simulink model "ThdRwRtStFwdBkwdTrgtPosSelc"  (R2018b)
settings: Solver=FixedStepDiscrete  StartTime=0.0  StopTime=10.0  FixedStep=0.01  RelTol=1e-3
undefined symbols (not defined in the file or in its folder): KeSMSw6sAcsEntryThdRwRtStFrwdBkwdPos_Val, KeSMSw6sAcsEntryThdRwRtStFrwdBkwdPosMax_Val, KeSMSw6sAcsEntryThdRwRtStFrwdBkwdPosMin_Val, KeSMSw6sFamilyMdThdRwRtStFrwdBkwdPos_Val, KeSMSw6sFamilyMdThdRwRtStFrwdBkwdPosMax_Val, KeSMSw6sFamilyMdThdRwRtStFrwdBkwdPosMin_Val, KeSMSw6sFamilyRMdThdRwRtStFrwdBkwdPos_Val, KeSMSw6sFamilyRMdThdRwRtStFrwdBkwdPosMax_Val, KeSMSw6sFamilyRMdThdRwRtStFrwdBkwdPosMin_Val, KeSMSw6sLugThdRwRtStFrwdBkwdPos_Val, KeSMSw6sLugThdRwRtStFrwdBkwdPosMax_Val, KeSMSw6sLugThdRwRtStFrwdBkwdPosMin_Val, KeSMSw6sVIPThdRwRtStFrwdBkwdPos_Val, KeSMSw6sVIPThdRwRtStFrwdBkwdPosMax_Val, KeSMSw6sVIPThdRwRtStFrwdBkwdPosMin_Val, KeSMSwAcsEntryThdRwRtStFrwdBkwdPos_Val, KeSMSwAcsEntryThdRwRtStFrwdBkwdPosMax_Val, KeSMSwAcsEntryThdRwRtStFrwdBkwdPosMin_Val, KeSMSwFamilyMdThdRwRtStFrwdBkwdPos_Val, KeSMSwFamilyMdThdRwRtStFrwdBkwdPosMax_Val, KeSMSwFamilyMdThdRwRtStFrwdBkwdPosMin_Val, KeSMSwFamilyRMdThdRwRtStFrwdBkwdPos_Val, KeSMSwFamilyRMdThdRwRtStFrwdBkwdPosMax_Val, KeSMSwFamilyRMdThdRwRtStFrwdBkwdPosMin_Val, KeSMSwLugThdRwRtStFrwdBkwdPos_Val, KeSMSwLugThdRwRtStFrwdBkwdPosMax_Val, KeSMSwLugThdRwRtStFrwdBkwdPosMin_Val, KeSMSwVIPThdRwRtStFrwdBkwdPos_Val, KeSMSwVIPThdRwRtStFrwdBkwdPosMax_Val, KeSMSwVIPThdRwRtStFrwdBkwdPosMin_Val
libraries: TrgtPosSelcLib x6
settings Model: Creator=sn2xws  LastModifiedBy=sn2xws
settings Model: ModifiedHistory=|
  | V2.1.0 Bug 540874 将外部标定改为固定值0
  | 2024.7.8 V3.0.0 557模式流程V1.9
settings DataIOCC: SaveFormat=StructureWithTime
settings OptimizationCC: DefaultParameterBehavior=Inlined  EnhancedBackFolding=on  PassReuseOutputArgsAs=Individual arguments  ZeroExternalMemoryAtStartup=off  ZeroInternalMemoryAtStartup=off  OptimizeBlockOrder=speed  DifferentSizesBufferReuse=on  OptimizationCustomize=off
settings DebuggingCC: ParameterTunabilityLossMsg=error
settings SFSimCC: MATLABDynamicMemAlloc=off
settings RTWCC: SystemTargetFile=autosar.tlc  GenCodeOnly=on  TemplateMakefile=ert_default_tmf  Description=AUTOSAR  GenerateReport=on  IncludeHyperlinkInReport=on  LaunchReport=on  GenerateTraceInfo=on  GenerateTraceReport=on  GenerateTraceReportSl=on  GenerateTraceReportSf=on  GenerateTraceReportEml=on  GenerateCodeMetricsReport=on
settings CodeAppCC: ForceParamTrailComments=on  IgnoreCustomStorageClasses=off  OperatorAnnotations=on  SimulinkDataObjDesc=on  SFDataObjDesc=on  InsertBlockDesc=on
settings STFCustomTargetCC: TargetLangStandard=C99 (ISO)  MultiwordLength=256  ParMdlRefBuildCompliant=on  CompOptLevelCompliant=on  IncludeMdlTerminateFcn=off  CombineOutputUpdateFcns=on  SuppressErrorStatus=on  ERTCustomFileBanners=on  SupportNonFinite=off  SupportComplex=off  SupportContinuousTime=off  SupportNonInlinedSFcns=off  RemoveResetFunc=on  MATLABClassNameForMDSCustomization=Simulink.SoftwareTarget.ERTCustomization  AutosarCompliant=on  UseToolchainInfoCompliant=on  LookupTableObjectStructAxisOrder=2,1,3,4,...  LUTObjectStructOrderEvenSpacing=Size,Table,Breakpoints  SystemTargetFile=autosar.tlc
settings ERTTargetCC: TargetLangStandard=C99 (ISO)  ConcurrentExecutionCompliant=off  IncludeMdlTerminateFcn=off  SuppressErrorStatus=on  SupportNonFinite=off  SupportComplex=off  ModelStepFunctionPrototypeControlCompliant=off  CPPClassGenCompliant=off  AutosarCompliant=on  LookupTableObjectStructAxisOrder=2,1,3,4,...  LUTObjectStructOrderEvenSpacing=Size,Table,Breakpoints  InlinedParameterPlacement=NonHierarchical  ERTCustomFileTemplate=example_file_process.tlc  ERTFilePackagingFormat=Compact

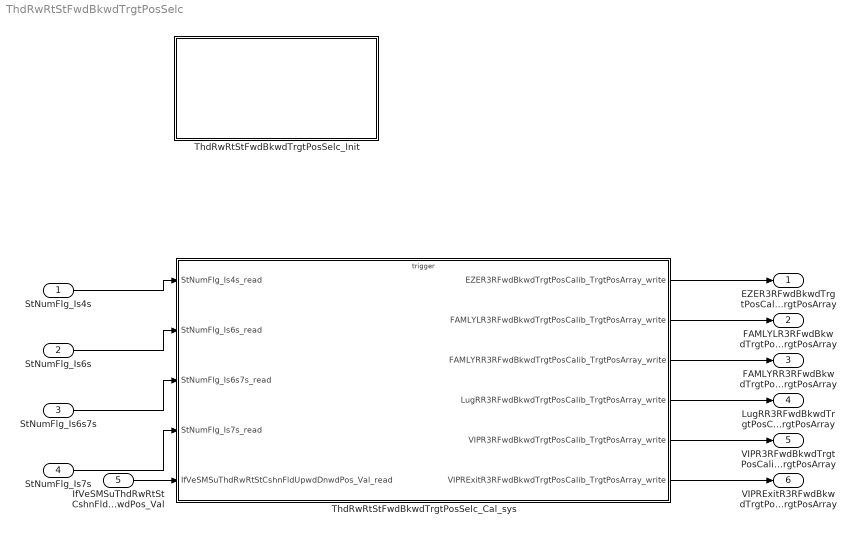
== system ThdRwRtStFwdBkwdTrgtPosSelc ==
  StNumFlg_Is4s : Inport  OutDataTypeStr=boolean  PortDimensions=1
  StNumFlg_Is6s : Inport  Port=2  OutDataTypeStr=boolean  PortDimensions=1
  StNumFlg_Is6s7s : Inport  Port=3  OutDataTypeStr=boolean  PortDimensions=1
  StNumFlg_Is7s : Inport  Port=4  OutDataTypeStr=boolean  PortDimensions=1
  IfVeSMSuThdRwRtStCshnFldUpwdDnwdPos_Val : Inport  Port=5  OutDataTypeStr=uint16  PortDimensions=1
  ThdRwRtStFwdBkwdTrgtPosSelc_Cal_sys : Subsystem
  ThdRwRtStFwdBkwdTrgtPosSelc_Init : Subsystem
  EZER3RFwdBkwdTrgtPosCalib_TrgtPosArray : Outport  Description=|  OutDataTypeStr=uint16  PortDimensions=3
      | 0:Pos
      | 1:Max
      | 2:Min
  FAMLYLR3RFwdBkwdTrgtPosCalib_TrgtPosArray : Outport  Description=|  Port=2  OutDataTypeStr=uint16  PortDimensions=3
      | 0:Pos
      | 1:Max
      | 2:Min
  FAMLYRR3RFwdBkwdTrgtPosCalib_TrgtPosArray : Outport  Description=|  Port=3  OutDataTypeStr=uint16  PortDimensions=3
      | 0:Pos
      | 1:Max
      | 2:Min
  LugRR3RFwdBkwdTrgtPosCalib_TrgtPosArray : Outport  Description=|  Port=4  OutDataTypeStr=uint16  PortDimensions=3
      | 0:Pos
      | 1:Max
      | 2:Min
  VIPR3RFwdBkwdTrgtPosCalib_TrgtPosArray : Outport  Description=|  Port=5  OutDataTypeStr=uint16  PortDimensions=3
      | 0:Pos
      | 1:Max
      | 2:Min
  VIPRExitR3RFwdBkwdTrgtPosCalib_TrgtPosArray : Outport  Description=|  Port=6  OutDataTypeStr=uint16  PortDimensions=3
      | 0:Pos
      | 1:Max
      | 2:Min
  wires:
  StNumFlg_Is4s/1 -> ThdRwRtStFwdBkwdTrgtPosSelc_Cal_sys/1(StNumFlg_Is4s_read)
  StNumFlg_Is6s/1 -> ThdRwRtStFwdBkwdTrgtPosSelc_Cal_sys/2(StNumFlg_Is6s_read)
  StNumFlg_Is6s7s/1 -> ThdRwRtStFwdBkwdTrgtPosSelc_Cal_sys/3(StNumFlg_Is6s7s_read)
  StNumFlg_Is7s/1 -> ThdRwRtStFwdBkwdTrgtPosSelc_Cal_sys/4(StNumFlg_Is7s_read)
  ThdRwRtStFwdBkwdTrgtPosSelc_Cal_sys/1(EZER3RFwdBkwdTrgtPosCalib_TrgtPosArray_write) -> EZER3RFwdBkwdTrgtPosCalib_TrgtPosArray/1
  ThdRwRtStFwdBkwdTrgtPosSelc_Cal_sys/2(FAMLYLR3RFwdBkwdTrgtPosCalib_TrgtPosArray_write) -> FAMLYLR3RFwdBkwdTrgtPosCalib_TrgtPosArray/1
  ThdRwRtStFwdBkwdTrgtPosSelc_Cal_sys/3(FAMLYRR3RFwdBkwdTrgtPosCalib_TrgtPosArray_write) -> FAMLYRR3RFwdBkwdTrgtPosCalib_TrgtPosArray/1
  ThdRwRtStFwdBkwdTrgtPosSelc_Cal_sys/4(LugRR3RFwdBkwdTrgtPosCalib_TrgtPosArray_write) -> LugRR3RFwdBkwdTrgtPosCalib_TrgtPosArray/1
  ThdRwRtStFwdBkwdTrgtPosSelc_Cal_sys/5(VIPR3RFwdBkwdTrgtPosCalib_TrgtPosArray_write) -> VIPR3RFwdBkwdTrgtPosCalib_TrgtPosArray/1
  ThdRwRtStFwdBkwdTrgtPosSelc_Cal_sys/6(VIPRExitR3RFwdBkwdTrgtPosCalib_TrgtPosArray_write) -> VIPRExitR3RFwdBkwdTrgtPosCalib_TrgtPosArray/1
  IfVeSMSuThdRwRtStCshnFldUpwdDnwdPos_Val/1 -> ThdRwRtStFwdBkwdTrgtPosSelc_Cal_sys/5(IfVeSMSuThdRwRtStCshnFldUpwdDnwdPos_Val_read)

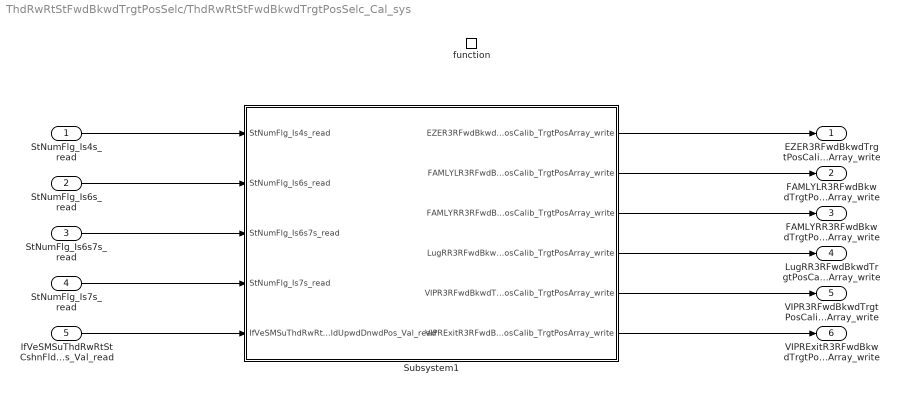
== system ThdRwRtStFwdBkwdTrgtPosSelc/ThdRwRtStFwdBkwdTrgtPosSelc_Cal_sys ==
  StNumFlg_Is4s_read : Inport
  StNumFlg_Is6s_read : Inport  Port=2
  StNumFlg_Is6s7s_read : Inport  Port=3
  StNumFlg_Is7s_read : Inport  Port=4
  IfVeSMSuThdRwRtStCshnFldUpwdDnwdPos_Val_read : Inport  Port=5
  function : TriggerPort  TriggerType=function-call  IsSimulinkFunction=on  FunctionName=ThdRwRtStFwdBkwdTrgtPosSelc_Cal  VariantControl=(inherit)
  Subsystem1 : Subsystem
  EZER3RFwdBkwdTrgtPosCalib_TrgtPosArray_write : Outport
      settings: EnsureOutportIsVirtual=on
  FAMLYLR3RFwdBkwdTrgtPosCalib_TrgtPosArray_write : Outport  Port=2
      settings: EnsureOutportIsVirtual=on
  FAMLYRR3RFwdBkwdTrgtPosCalib_TrgtPosArray_write : Outport  Port=3
      settings: EnsureOutportIsVirtual=on
  LugRR3RFwdBkwdTrgtPosCalib_TrgtPosArray_write : Outport  Port=4
      settings: EnsureOutportIsVirtual=on
  VIPR3RFwdBkwdTrgtPosCalib_TrgtPosArray_write : Outport  Port=5
      settings: EnsureOutportIsVirtual=on
  VIPRExitR3RFwdBkwdTrgtPosCalib_TrgtPosArray_write : Outport  Port=6
      settings: EnsureOutportIsVirtual=on
  wires:
  Subsystem1/2(FAMLYLR3RFwdBkwdTrgtPosCalib_TrgtPosArray_write) -> FAMLYLR3RFwdBkwdTrgtPosCalib_TrgtPosArray_write/1
  Subsystem1/1(EZER3RFwdBkwdTrgtPosCalib_TrgtPosArray_write) -> EZER3RFwdBkwdTrgtPosCalib_TrgtPosArray_write/1
  Subsystem1/3(FAMLYRR3RFwdBkwdTrgtPosCalib_TrgtPosArray_write) -> FAMLYRR3RFwdBkwdTrgtPosCalib_TrgtPosArray_write/1
  Subsystem1/4(LugRR3RFwdBkwdTrgtPosCalib_TrgtPosArray_write) -> LugRR3RFwdBkwdTrgtPosCalib_TrgtPosArray_write/1
  Subsystem1/5(VIPR3RFwdBkwdTrgtPosCalib_TrgtPosArray_write) -> VIPR3RFwdBkwdTrgtPosCalib_TrgtPosArray_write/1
  StNumFlg_Is4s_read/1 -> Subsystem1/1(StNumFlg_Is4s_read)
  StNumFlg_Is6s_read/1 -> Subsystem1/2(StNumFlg_Is6s_read)
  StNumFlg_Is6s7s_read/1 -> Subsystem1/3(StNumFlg_Is6s7s_read)
  StNumFlg_Is7s_read/1 -> Subsystem1/4(StNumFlg_Is7s_read)
  Subsystem1/6(VIPRExitR3RFwdBkwdTrgtPosCalib_TrgtPosArray_write) -> VIPRExitR3RFwdBkwdTrgtPosCalib_TrgtPosArray_write/1
  IfVeSMSuThdRwRtStCshnFldUpwdDnwdPos_Val_read/1 -> Subsystem1/5(IfVeSMSuThdRwRtStCshnFldUpwdDnwdPos_Val_read)

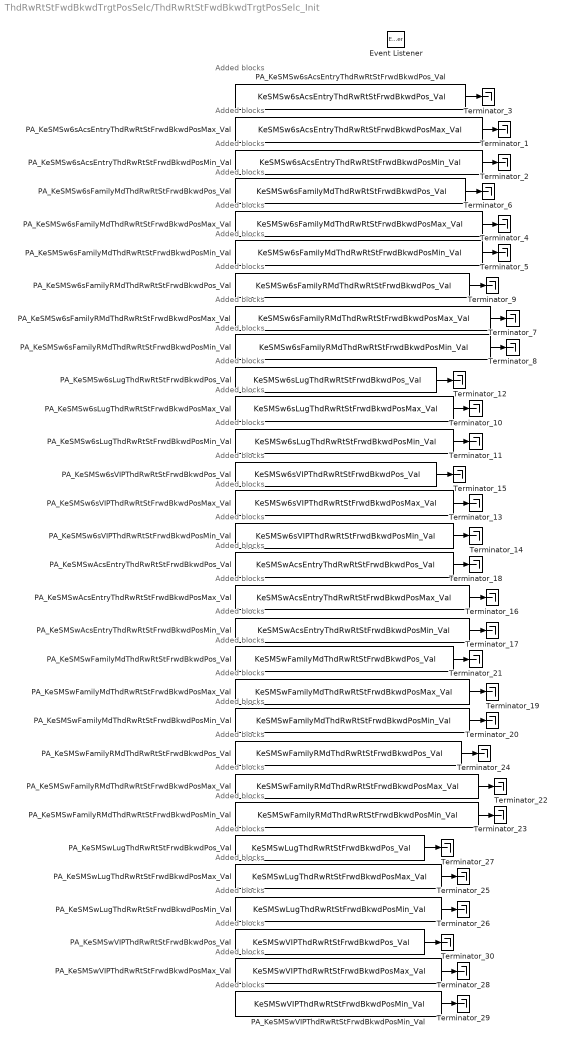
== system ThdRwRtStFwdBkwdTrgtPosSelc/ThdRwRtStFwdBkwdTrgtPosSelc_Init ==
  note: Added blocks
  note: Added blocks
  note: Added blocks
  note: Added blocks
  note: Added blocks
  note: Added blocks
  note: Added blocks
  note: Added blocks
  note: Added blocks
  note: Added blocks
  note: Added blocks
  note: Added blocks
  note: Added blocks
  note: Added blocks
  note: Added blocks
  note: Added blocks
  note: Added blocks
  note: Added blocks
  note: Added blocks
  note: Added blocks
  note: Added blocks
  note: Added blocks
  note: Added blocks
  note: Added blocks
  note: Added blocks
  note: Added blocks
  note: Added blocks
  note: Added blocks
  note: Added blocks
  note: Added blocks
  Event Listener : EventListener  EventName=reset
  PA_KeSMSw6sAcsEntryThdRwRtStFrwdBkwdPosMax_Val : Constant  Value=KeSMSw6sAcsEntryThdRwRtStFrwdBkwdPosMax_Val
  PA_KeSMSw6sAcsEntryThdRwRtStFrwdBkwdPosMin_Val : Constant  Value=KeSMSw6sAcsEntryThdRwRtStFrwdBkwdPosMin_Val
  PA_KeSMSw6sAcsEntryThdRwRtStFrwdBkwdPos_Val : Constant  Value=KeSMSw6sAcsEntryThdRwRtStFrwdBkwdPos_Val
  PA_KeSMSw6sFamilyMdThdRwRtStFrwdBkwdPosMax_Val : Constant  Value=KeSMSw6sFamilyMdThdRwRtStFrwdBkwdPosMax_Val
  PA_KeSMSw6sFamilyMdThdRwRtStFrwdBkwdPosMin_Val : Constant  Value=KeSMSw6sFamilyMdThdRwRtStFrwdBkwdPosMin_Val
  PA_KeSMSw6sFamilyMdThdRwRtStFrwdBkwdPos_Val : Constant  Value=KeSMSw6sFamilyMdThdRwRtStFrwdBkwdPos_Val
  PA_KeSMSw6sFamilyRMdThdRwRtStFrwdBkwdPosMax_Val : Constant  Value=KeSMSw6sFamilyRMdThdRwRtStFrwdBkwdPosMax_Val
  PA_KeSMSw6sFamilyRMdThdRwRtStFrwdBkwdPosMin_Val : Constant  Value=KeSMSw6sFamilyRMdThdRwRtStFrwdBkwdPosMin_Val
  PA_KeSMSw6sFamilyRMdThdRwRtStFrwdBkwdPos_Val : Constant  Value=KeSMSw6sFamilyRMdThdRwRtStFrwdBkwdPos_Val
  PA_KeSMSw6sLugThdRwRtStFrwdBkwdPosMax_Val : Constant  Value=KeSMSw6sLugThdRwRtStFrwdBkwdPosMax_Val
  PA_KeSMSw6sLugThdRwRtStFrwdBkwdPosMin_Val : Constant  Value=KeSMSw6sLugThdRwRtStFrwdBkwdPosMin_Val
  PA_KeSMSw6sLugThdRwRtStFrwdBkwdPos_Val : Constant  Value=KeSMSw6sLugThdRwRtStFrwdBkwdPos_Val
  PA_KeSMSw6sVIPThdRwRtStFrwdBkwdPosMax_Val : Constant  Value=KeSMSw6sVIPThdRwRtStFrwdBkwdPosMax_Val
  PA_KeSMSw6sVIPThdRwRtStFrwdBkwdPosMin_Val : Constant  Value=KeSMSw6sVIPThdRwRtStFrwdBkwdPosMin_Val
  PA_KeSMSw6sVIPThdRwRtStFrwdBkwdPos_Val : Constant  Value=KeSMSw6sVIPThdRwRtStFrwdBkwdPos_Val
  PA_KeSMSwAcsEntryThdRwRtStFrwdBkwdPosMax_Val : Constant  Value=KeSMSwAcsEntryThdRwRtStFrwdBkwdPosMax_Val
  PA_KeSMSwAcsEntryThdRwRtStFrwdBkwdPosMin_Val : Constant  Value=KeSMSwAcsEntryThdRwRtStFrwdBkwdPosMin_Val
  PA_KeSMSwAcsEntryThdRwRtStFrwdBkwdPos_Val : Constant  Value=KeSMSwAcsEntryThdRwRtStFrwdBkwdPos_Val
  PA_KeSMSwFamilyMdThdRwRtStFrwdBkwdPosMax_Val : Constant  Value=KeSMSwFamilyMdThdRwRtStFrwdBkwdPosMax_Val
  PA_KeSMSwFamilyMdThdRwRtStFrwdBkwdPosMin_Val : Constant  Value=KeSMSwFamilyMdThdRwRtStFrwdBkwdPosMin_Val
  PA_KeSMSwFamilyMdThdRwRtStFrwdBkwdPos_Val : Constant  Value=KeSMSwFamilyMdThdRwRtStFrwdBkwdPos_Val
  PA_KeSMSwFamilyRMdThdRwRtStFrwdBkwdPosMax_Val : Constant  Value=KeSMSwFamilyRMdThdRwRtStFrwdBkwdPosMax_Val
  PA_KeSMSwFamilyRMdThdRwRtStFrwdBkwdPosMin_Val : Constant  Value=KeSMSwFamilyRMdThdRwRtStFrwdBkwdPosMin_Val
  PA_KeSMSwFamilyRMdThdRwRtStFrwdBkwdPos_Val : Constant  Value=KeSMSwFamilyRMdThdRwRtStFrwdBkwdPos_Val
  PA_KeSMSwLugThdRwRtStFrwdBkwdPosMax_Val : Constant  Value=KeSMSwLugThdRwRtStFrwdBkwdPosMax_Val
  PA_KeSMSwLugThdRwRtStFrwdBkwdPosMin_Val : Constant  Value=KeSMSwLugThdRwRtStFrwdBkwdPosMin_Val
  PA_KeSMSwLugThdRwRtStFrwdBkwdPos_Val : Constant  Value=KeSMSwLugThdRwRtStFrwdBkwdPos_Val
  PA_KeSMSwVIPThdRwRtStFrwdBkwdPosMax_Val : Constant  Value=KeSMSwVIPThdRwRtStFrwdBkwdPosMax_Val
  PA_KeSMSwVIPThdRwRtStFrwdBkwdPosMin_Val : Constant  Value=KeSMSwVIPThdRwRtStFrwdBkwdPosMin_Val
  PA_KeSMSwVIPThdRwRtStFrwdBkwdPos_Val : Constant  Value=KeSMSwVIPThdRwRtStFrwdBkwdPos_Val
  Terminator_{1..30} (30 alike) : Terminator
  wires:
  PA_KeSMSw6sAcsEntryThdRwRtStFrwdBkwdPosMax_Val/1 -> Terminator_1/1
  PA_KeSMSw6sAcsEntryThdRwRtStFrwdBkwdPosMin_Val/1 -> Terminator_2/1
  PA_KeSMSw6sAcsEntryThdRwRtStFrwdBkwdPos_Val/1 -> Terminator_3/1
  PA_KeSMSw6sFamilyMdThdRwRtStFrwdBkwdPosMax_Val/1 -> Terminator_4/1
  PA_KeSMSw6sFamilyMdThdRwRtStFrwdBkwdPosMin_Val/1 -> Terminator_5/1
  PA_KeSMSw6sFamilyMdThdRwRtStFrwdBkwdPos_Val/1 -> Terminator_6/1
  PA_KeSMSw6sFamilyRMdThdRwRtStFrwdBkwdPosMax_Val/1 -> Terminator_7/1
  PA_KeSMSw6sFamilyRMdThdRwRtStFrwdBkwdPosMin_Val/1 -> Terminator_8/1
  PA_KeSMSw6sFamilyRMdThdRwRtStFrwdBkwdPos_Val/1 -> Terminator_9/1
  PA_KeSMSw6sLugThdRwRtStFrwdBkwdPosMax_Val/1 -> Terminator_10/1
  PA_KeSMSw6sLugThdRwRtStFrwdBkwdPosMin_Val/1 -> Terminator_11/1
  PA_KeSMSw6sLugThdRwRtStFrwdBkwdPos_Val/1 -> Terminator_12/1
  PA_KeSMSw6sVIPThdRwRtStFrwdBkwdPosMax_Val/1 -> Terminator_13/1
  PA_KeSMSw6sVIPThdRwRtStFrwdBkwdPosMin_Val/1 -> Terminator_14/1
  PA_KeSMSw6sVIPThdRwRtStFrwdBkwdPos_Val/1 -> Terminator_15/1
  PA_KeSMSwAcsEntryThdRwRtStFrwdBkwdPosMax_Val/1 -> Terminator_16/1
  PA_KeSMSwAcsEntryThdRwRtStFrwdBkwdPosMin_Val/1 -> Terminator_17/1
  PA_KeSMSwAcsEntryThdRwRtStFrwdBkwdPos_Val/1 -> Terminator_18/1
  PA_KeSMSwFamilyMdThdRwRtStFrwdBkwdPosMax_Val/1 -> Terminator_19/1
  PA_KeSMSwFamilyMdThdRwRtStFrwdBkwdPosMin_Val/1 -> Terminator_20/1
  PA_KeSMSwFamilyMdThdRwRtStFrwdBkwdPos_Val/1 -> Terminator_21/1
  PA_KeSMSwFamilyRMdThdRwRtStFrwdBkwdPosMax_Val/1 -> Terminator_22/1
  PA_KeSMSwFamilyRMdThdRwRtStFrwdBkwdPosMin_Val/1 -> Terminator_23/1
  PA_KeSMSwFamilyRMdThdRwRtStFrwdBkwdPos_Val/1 -> Terminator_24/1
  PA_KeSMSwLugThdRwRtStFrwdBkwdPosMax_Val/1 -> Terminator_25/1
  PA_KeSMSwLugThdRwRtStFrwdBkwdPosMin_Val/1 -> Terminator_26/1
  PA_KeSMSwLugThdRwRtStFrwdBkwdPos_Val/1 -> Terminator_27/1
  PA_KeSMSwVIPThdRwRtStFrwdBkwdPosMax_Val/1 -> Terminator_28/1
  PA_KeSMSwVIPThdRwRtStFrwdBkwdPosMin_Val/1 -> Terminator_29/1
  PA_KeSMSwVIPThdRwRtStFrwdBkwdPos_Val/1 -> Terminator_30/1

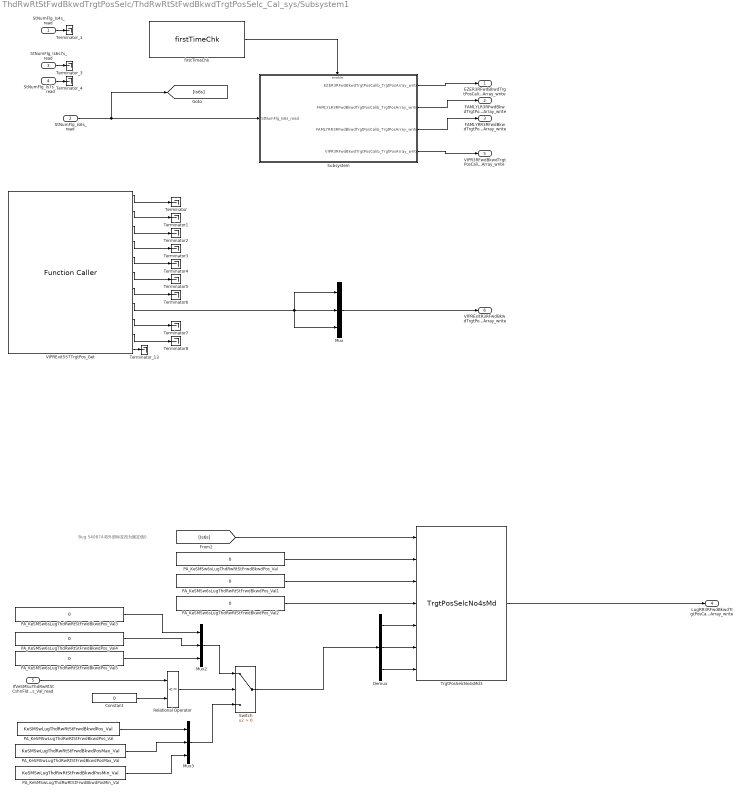
== system ThdRwRtStFwdBkwdTrgtPosSelc/ThdRwRtStFwdBkwdTrgtPosSelc_Cal_sys/Subsystem1 ==
  note: Bug 540874 将外部标定改为固定值0
  StNumFlg_Is4s_read : Inport
  StNumFlg_Is6s_read : Inport  Port=2
  StNumFlg_Is6s7s_read : Inport  Port=3
  StNumFlg_Is7s_read : Inport  Port=4
  IfVeSMSuThdRwRtStCshnFldUpwdDnwdPos_Val_read : Inport  Port=5
  Constant : Constant  Value=0  OutDataTypeStr=uint16
  Demux : Demux  Outputs=3
  Mux : Mux  Inputs=3
  Mux2 : Mux  Inputs=3
  Mux3 : Mux  Inputs=3
  PA_KeSMSw6sLugThdRwRtStFrwdBkwdPos_Val{,1..5} (6 alike) : Constant  Value=0  OutDataTypeStr=uint16
  PA_KeSMSwLugThdRwRtStFrwdBkwdPosMax_Val : Constant  Value=KeSMSwLugThdRwRtStFrwdBkwdPosMax_Val
  PA_KeSMSwLugThdRwRtStFrwdBkwdPosMin_Val : Constant  Value=KeSMSwLugThdRwRtStFrwdBkwdPosMin_Val
  PA_KeSMSwLugThdRwRtStFrwdBkwdPos_Val : Constant  Value=KeSMSwLugThdRwRtStFrwdBkwdPos_Val
  Relational Operator : RelationalOperator  Operator=<=  OutDataTypeStr=boolean  RndMeth=Simplest
  Subsystem : Subsystem
  Switch : Switch  Criteria=u2 > Threshold
  Terminator{,1..8} (9 alike) : Terminator
  Terminator_{1,3..4,13} (4 alike) : Terminator
  TrgtPosSelcNo4sMd3 : TrgtPosSelcLib/TrgtPosSelcNo4sMd  SystemSampleTime=-1
  VIPRExit557TrgtPos_Get : FunctionCaller  FunctionPrototype=[SecRwRtStBkReclnTrgtPos,SecRwRtStZeroTrgtPos,SecRwRtStLgrstUpwdDnwdTrgtPos,SecRwRtStLgrstInwdOtwdTrgtPos,ThdRwLtStBkReclnTrgtPos,ThdRwLtStFwdBkwdTrgtPos,ThdRwRtStBkReclnTrgtPos,ThdRwRtStFwdBkwdTrgtPos,PassStBkReclnTrgtPos,PassStFwdBkwdTrgtPos,SecRwRtStFwdBkwdTrgtPos] = VIPRExit557TrgtPos_Get()  OutputArgumentSpecifications=uint16(1), uint16(1), uint16(1), uint16(1), uint16(1), uint16(1), uint16(1), uint16(1), uint16(1), uint16(1), uint16(1)
  firstTimeChk : TrgtPosSelcLib/firstTimeChk  SystemSampleTime=-1
  EZER3RFwdBkwdTrgtPosCalib_TrgtPosArray_write : Outport
      settings: EnsureOutportIsVirtual=on
  FAMLYLR3RFwdBkwdTrgtPosCalib_TrgtPosArray_write : Outport  Port=2
      settings: EnsureOutportIsVirtual=on
  FAMLYRR3RFwdBkwdTrgtPosCalib_TrgtPosArray_write : Outport  Port=3
      settings: EnsureOutportIsVirtual=on
  LugRR3RFwdBkwdTrgtPosCalib_TrgtPosArray_write : Outport  Port=4
      settings: EnsureOutportIsVirtual=on
  VIPR3RFwdBkwdTrgtPosCalib_TrgtPosArray_write : Outport  Port=5
      settings: EnsureOutportIsVirtual=on
  VIPRExitR3RFwdBkwdTrgtPosCalib_TrgtPosArray_write : Outport  Port=6
      settings: EnsureOutportIsVirtual=on
  wires:
  StNumFlg_Is6s7s_read/1 -> Terminator_3/1
  StNumFlg_Is7s_read/1 -> Terminator_4/1
  Subsystem/4(VIPR3RFwdBkwdTrgtPosCalib_TrgtPosArray_write) -> VIPR3RFwdBkwdTrgtPosCalib_TrgtPosArray_write/1
  Subsystem/2(FAMLYLR3RFwdBkwdTrgtPosCalib_TrgtPosArray_write) -> FAMLYLR3RFwdBkwdTrgtPosCalib_TrgtPosArray_write/1
  StNumFlg_Is4s_read/1 -> Terminator_1/1
  Subsystem/3(FAMLYRR3RFwdBkwdTrgtPosCalib_TrgtPosArray_write) -> FAMLYRR3RFwdBkwdTrgtPosCalib_TrgtPosArray_write/1
  firstTimeChk/1 -> Subsystem/Enable
  StNumFlg_Is6s_read/1 -> [Is6s], Subsystem/1(StNumFlg_Is6s_read)
  TrgtPosSelcNo4sMd3/1 -> LugRR3RFwdBkwdTrgtPosCalib_TrgtPosArray_write/1
  Subsystem/1(EZER3RFwdBkwdTrgtPosCalib_TrgtPosArray_write) -> EZER3RFwdBkwdTrgtPosCalib_TrgtPosArray_write/1
  VIPRExit557TrgtPos_Get/1 -> Terminator/1
  VIPRExit557TrgtPos_Get/2 -> Terminator1/1
  VIPRExit557TrgtPos_Get/3 -> Terminator2/1
  VIPRExit557TrgtPos_Get/4 -> Terminator3/1
  VIPRExit557TrgtPos_Get/5 -> Terminator4/1
  VIPRExit557TrgtPos_Get/6 -> Terminator5/1
  VIPRExit557TrgtPos_Get/7 -> Terminator6/1
  VIPRExit557TrgtPos_Get/9 -> Terminator7/1
  VIPRExit557TrgtPos_Get/10 -> Terminator8/1
  Mux/1 -> VIPRExitR3RFwdBkwdTrgtPosCalib_TrgtPosArray_write/1
  VIPRExit557TrgtPos_Get/8 -> Mux/2, Mux/3, Mux/1
  VIPRExit557TrgtPos_Get/11 -> Terminator_13/1
  [Is6s] -> TrgtPosSelcNo4sMd3/1
  PA_KeSMSw6sLugThdRwRtStFrwdBkwdPos_Val1/1 -> TrgtPosSelcNo4sMd3/3
  PA_KeSMSw6sLugThdRwRtStFrwdBkwdPos_Val2/1 -> TrgtPosSelcNo4sMd3/4
  PA_KeSMSw6sLugThdRwRtStFrwdBkwdPos_Val/1 -> TrgtPosSelcNo4sMd3/2
  PA_KeSMSwLugThdRwRtStFrwdBkwdPos_Val/1 -> Mux3/1
  Demux/1 -> TrgtPosSelcNo4sMd3/5
  PA_KeSMSw6sLugThdRwRtStFrwdBkwdPos_Val4/1 -> Mux2/2
  Switch/1 -> Demux/1
  Mux3/1 -> Switch/3
  PA_KeSMSwLugThdRwRtStFrwdBkwdPosMin_Val/1 -> Mux3/3
  Mux2/1 -> Switch/1
  Relational Operator/1 -> Switch/2
  PA_KeSMSw6sLugThdRwRtStFrwdBkwdPos_Val5/1 -> Mux2/3
  Demux/3 -> TrgtPosSelcNo4sMd3/7
  PA_KeSMSwLugThdRwRtStFrwdBkwdPosMax_Val/1 -> Mux3/2
  PA_KeSMSw6sLugThdRwRtStFrwdBkwdPos_Val3/1 -> Mux2/1
  Demux/2 -> TrgtPosSelcNo4sMd3/6
  IfVeSMSuThdRwRtStCshnFldUpwdDnwdPos_Val_read/1 -> Relational Operator/1
  Constant/1 -> Relational Operator/2

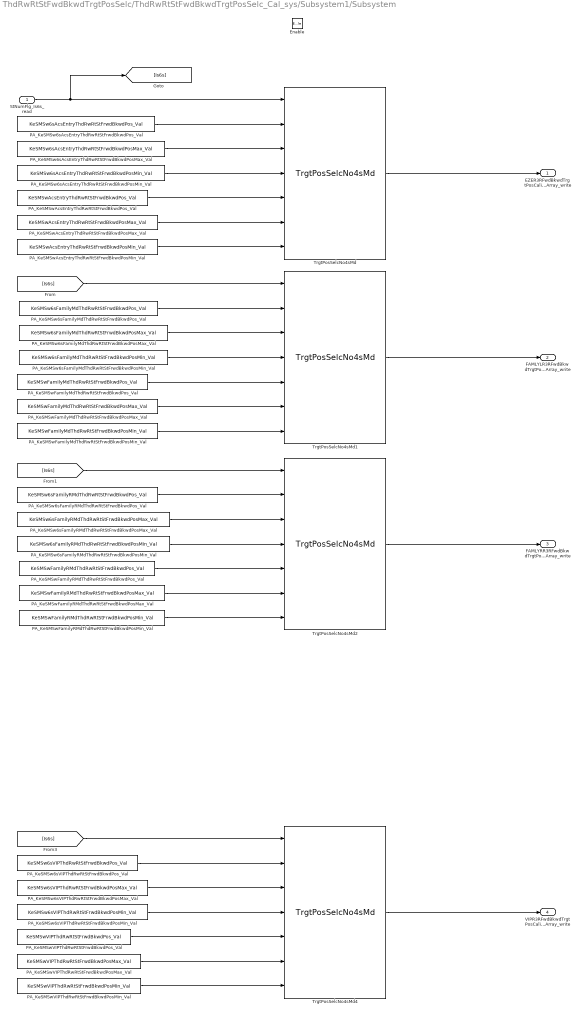
== system ThdRwRtStFwdBkwdTrgtPosSelc/ThdRwRtStFwdBkwdTrgtPosSelc_Cal_sys/Subsystem1/Subsystem ==
  StNumFlg_Is6s_read : Inport
  Enable : EnablePort
  PA_KeSMSw6sAcsEntryThdRwRtStFrwdBkwdPosMax_Val : Constant  Value=KeSMSw6sAcsEntryThdRwRtStFrwdBkwdPosMax_Val
  PA_KeSMSw6sAcsEntryThdRwRtStFrwdBkwdPosMin_Val : Constant  Value=KeSMSw6sAcsEntryThdRwRtStFrwdBkwdPosMin_Val
  PA_KeSMSw6sAcsEntryThdRwRtStFrwdBkwdPos_Val : Constant  Value=KeSMSw6sAcsEntryThdRwRtStFrwdBkwdPos_Val
  PA_KeSMSw6sFamilyMdThdRwRtStFrwdBkwdPosMax_Val : Constant  Value=KeSMSw6sFamilyMdThdRwRtStFrwdBkwdPosMax_Val
  PA_KeSMSw6sFamilyMdThdRwRtStFrwdBkwdPosMin_Val : Constant  Value=KeSMSw6sFamilyMdThdRwRtStFrwdBkwdPosMin_Val
  PA_KeSMSw6sFamilyMdThdRwRtStFrwdBkwdPos_Val : Constant  Value=KeSMSw6sFamilyMdThdRwRtStFrwdBkwdPos_Val
  PA_KeSMSw6sFamilyRMdThdRwRtStFrwdBkwdPosMax_Val : Constant  Value=KeSMSw6sFamilyRMdThdRwRtStFrwdBkwdPosMax_Val
  PA_KeSMSw6sFamilyRMdThdRwRtStFrwdBkwdPosMin_Val : Constant  Value=KeSMSw6sFamilyRMdThdRwRtStFrwdBkwdPosMin_Val
  PA_KeSMSw6sFamilyRMdThdRwRtStFrwdBkwdPos_Val : Constant  Value=KeSMSw6sFamilyRMdThdRwRtStFrwdBkwdPos_Val
  PA_KeSMSw6sVIPThdRwRtStFrwdBkwdPosMax_Val : Constant  Value=KeSMSw6sVIPThdRwRtStFrwdBkwdPosMax_Val
  PA_KeSMSw6sVIPThdRwRtStFrwdBkwdPosMin_Val : Constant  Value=KeSMSw6sVIPThdRwRtStFrwdBkwdPosMin_Val
  PA_KeSMSw6sVIPThdRwRtStFrwdBkwdPos_Val : Constant  Value=KeSMSw6sVIPThdRwRtStFrwdBkwdPos_Val
  PA_KeSMSwAcsEntryThdRwRtStFrwdBkwdPosMax_Val : Constant  Value=KeSMSwAcsEntryThdRwRtStFrwdBkwdPosMax_Val
  PA_KeSMSwAcsEntryThdRwRtStFrwdBkwdPosMin_Val : Constant  Value=KeSMSwAcsEntryThdRwRtStFrwdBkwdPosMin_Val
  PA_KeSMSwAcsEntryThdRwRtStFrwdBkwdPos_Val : Constant  Value=KeSMSwAcsEntryThdRwRtStFrwdBkwdPos_Val
  PA_KeSMSwFamilyMdThdRwRtStFrwdBkwdPosMax_Val : Constant  Value=KeSMSwFamilyMdThdRwRtStFrwdBkwdPosMax_Val
  PA_KeSMSwFamilyMdThdRwRtStFrwdBkwdPosMin_Val : Constant  Value=KeSMSwFamilyMdThdRwRtStFrwdBkwdPosMin_Val
  PA_KeSMSwFamilyMdThdRwRtStFrwdBkwdPos_Val : Constant  Value=KeSMSwFamilyMdThdRwRtStFrwdBkwdPos_Val
  PA_KeSMSwFamilyRMdThdRwRtStFrwdBkwdPosMax_Val : Constant  Value=KeSMSwFamilyRMdThdRwRtStFrwdBkwdPosMax_Val
  PA_KeSMSwFamilyRMdThdRwRtStFrwdBkwdPosMin_Val : Constant  Value=KeSMSwFamilyRMdThdRwRtStFrwdBkwdPosMin_Val
  PA_KeSMSwFamilyRMdThdRwRtStFrwdBkwdPos_Val : Constant  Value=KeSMSwFamilyRMdThdRwRtStFrwdBkwdPos_Val
  PA_KeSMSwVIPThdRwRtStFrwdBkwdPosMax_Val : Constant  Value=KeSMSwVIPThdRwRtStFrwdBkwdPosMax_Val
  PA_KeSMSwVIPThdRwRtStFrwdBkwdPosMin_Val : Constant  Value=KeSMSwVIPThdRwRtStFrwdBkwdPosMin_Val
  PA_KeSMSwVIPThdRwRtStFrwdBkwdPos_Val : Constant  Value=KeSMSwVIPThdRwRtStFrwdBkwdPos_Val
  TrgtPosSelcNo4sMd{,1..2,4} (4 alike) : TrgtPosSelcLib/TrgtPosSelcNo4sMd  SystemSampleTime=-1
  EZER3RFwdBkwdTrgtPosCalib_TrgtPosArray_write : Outport
      settings: EnsureOutportIsVirtual=on
  FAMLYLR3RFwdBkwdTrgtPosCalib_TrgtPosArray_write : Outport  Port=2
      settings: EnsureOutportIsVirtual=on
  FAMLYRR3RFwdBkwdTrgtPosCalib_TrgtPosArray_write : Outport  Port=3
      settings: EnsureOutportIsVirtual=on
  VIPR3RFwdBkwdTrgtPosCalib_TrgtPosArray_write : Outport  Port=4
      settings: EnsureOutportIsVirtual=on
  wires:
  StNumFlg_Is6s_read/1 -> [Is6s], TrgtPosSelcNo4sMd/1
  [Is6s] -> TrgtPosSelcNo4sMd1/1
  [Is6s] -> TrgtPosSelcNo4sMd2/1
  [Is6s] -> TrgtPosSelcNo4sMd4/1
  PA_KeSMSw6sAcsEntryThdRwRtStFrwdBkwdPosMax_Val/1 -> TrgtPosSelcNo4sMd/3
  PA_KeSMSw6sAcsEntryThdRwRtStFrwdBkwdPos_Val/1 -> TrgtPosSelcNo4sMd/2
  PA_KeSMSw6sAcsEntryThdRwRtStFrwdBkwdPosMin_Val/1 -> TrgtPosSelcNo4sMd/4
  PA_KeSMSw6sFamilyMdThdRwRtStFrwdBkwdPosMax_Val/1 -> TrgtPosSelcNo4sMd1/3
  PA_KeSMSw6sFamilyMdThdRwRtStFrwdBkwdPos_Val/1 -> TrgtPosSelcNo4sMd1/2
  PA_KeSMSw6sFamilyMdThdRwRtStFrwdBkwdPosMin_Val/1 -> TrgtPosSelcNo4sMd1/4
  PA_KeSMSw6sFamilyRMdThdRwRtStFrwdBkwdPosMax_Val/1 -> TrgtPosSelcNo4sMd2/3
  PA_KeSMSw6sFamilyRMdThdRwRtStFrwdBkwdPosMin_Val/1 -> TrgtPosSelcNo4sMd2/4
  PA_KeSMSw6sFamilyRMdThdRwRtStFrwdBkwdPos_Val/1 -> TrgtPosSelcNo4sMd2/2
  PA_KeSMSw6sVIPThdRwRtStFrwdBkwdPosMax_Val/1 -> TrgtPosSelcNo4sMd4/3
  PA_KeSMSw6sVIPThdRwRtStFrwdBkwdPos_Val/1 -> TrgtPosSelcNo4sMd4/2
  PA_KeSMSw6sVIPThdRwRtStFrwdBkwdPosMin_Val/1 -> TrgtPosSelcNo4sMd4/4
  PA_KeSMSwAcsEntryThdRwRtStFrwdBkwdPosMax_Val/1 -> TrgtPosSelcNo4sMd/6
  PA_KeSMSwAcsEntryThdRwRtStFrwdBkwdPos_Val/1 -> TrgtPosSelcNo4sMd/5
  PA_KeSMSwAcsEntryThdRwRtStFrwdBkwdPosMin_Val/1 -> TrgtPosSelcNo4sMd/7
  PA_KeSMSwFamilyMdThdRwRtStFrwdBkwdPosMax_Val/1 -> TrgtPosSelcNo4sMd1/6
  PA_KeSMSwFamilyMdThdRwRtStFrwdBkwdPos_Val/1 -> TrgtPosSelcNo4sMd1/5
  PA_KeSMSwFamilyMdThdRwRtStFrwdBkwdPosMin_Val/1 -> TrgtPosSelcNo4sMd1/7
  PA_KeSMSwFamilyRMdThdRwRtStFrwdBkwdPosMax_Val/1 -> TrgtPosSelcNo4sMd2/6
  PA_KeSMSwFamilyRMdThdRwRtStFrwdBkwdPos_Val/1 -> TrgtPosSelcNo4sMd2/5
  PA_KeSMSwFamilyRMdThdRwRtStFrwdBkwdPosMin_Val/1 -> TrgtPosSelcNo4sMd2/7
  PA_KeSMSwVIPThdRwRtStFrwdBkwdPosMax_Val/1 -> TrgtPosSelcNo4sMd4/6
  PA_KeSMSwVIPThdRwRtStFrwdBkwdPos_Val/1 -> TrgtPosSelcNo4sMd4/5
  PA_KeSMSwVIPThdRwRtStFrwdBkwdPosMin_Val/1 -> TrgtPosSelcNo4sMd4/7
  TrgtPosSelcNo4sMd/1 -> EZER3RFwdBkwdTrgtPosCalib_TrgtPosArray_write/1
  TrgtPosSelcNo4sMd1/1 -> FAMLYLR3RFwdBkwdTrgtPosCalib_TrgtPosArray_write/1
  TrgtPosSelcNo4sMd2/1 -> FAMLYRR3RFwdBkwdTrgtPosCalib_TrgtPosArray_write/1
  TrgtPosSelcNo4sMd4/1 -> VIPR3RFwdBkwdTrgtPosCalib_TrgtPosArray_write/1
